simulink model "RoboticArmSimulation"  (R2025b)
settings: Solver=ode4  StartTime=0.0  StopTime=10  FixedStep=0.001  RelTol=1e-3
settings Model: Creator=james  LastModifiedBy=james

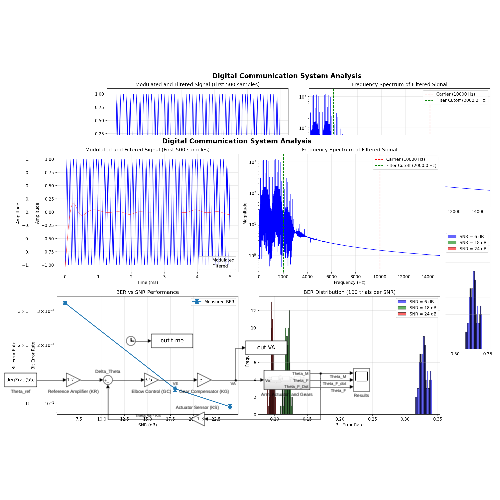
[thumbnail: Simulink's stored preview of the top-level diagram]
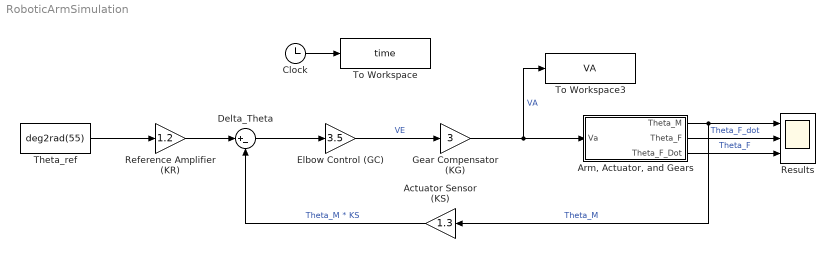
== system RoboticArmSimulation ==
  Actuator Sensor (KS) : Gain  Gain=1.3
  "Arm, Actuator, and Gears" : Subsystem
  Clock : Clock
  Delta_Theta : Sum  Inputs=|+-
  Elbow Control (GC) : Gain  Gain=3.5
  Gear Compensator (KG) : Gain  Gain=3
  Reference Amplifier (KR) : Gain  Gain=1.2
  Results : Scope  NumInputPorts=3
      settings: ActiveDisplayYMinimum=-2.9473768605800479  ActiveDisplayYMaximum=9.0057480309886788
  Theta_ref : Constant  Value=deg2rad(55)
  To Workspace : ToWorkspace  VariableName=time  SaveFormat=Timeseries  SampleTime=-1
  To Workspace3 : ToWorkspace  VariableName=VA  SaveFormat=Timeseries  SampleTime=-1
  wires:
  Theta_ref/1 -> Reference Amplifier (KR)/1
  Reference Amplifier (KR)/1 -> Delta_Theta/1
  Delta_Theta/1 -> Elbow Control (GC)/1
  Clock/1 -> To Workspace/1
  Elbow Control (GC)/1 -> Gear Compensator (KG)/1  "VE"
  Gear Compensator (KG)/1 -> To Workspace3/1, "Arm, Actuator, and Gears"/1(Va)  "VA"
  "Arm, Actuator, and Gears"/1(Theta_M) -> Actuator Sensor (KS)/1, Results/1  "Theta_M"
  "Arm, Actuator, and Gears"/2(Theta_F) -> Results/2  "Theta_F_dot"
  "Arm, Actuator, and Gears"/3(Theta_F_Dot) -> Results/3  "Theta_F"
  Actuator Sensor (KS)/1 -> Delta_Theta/2  "Theta_M * KS"

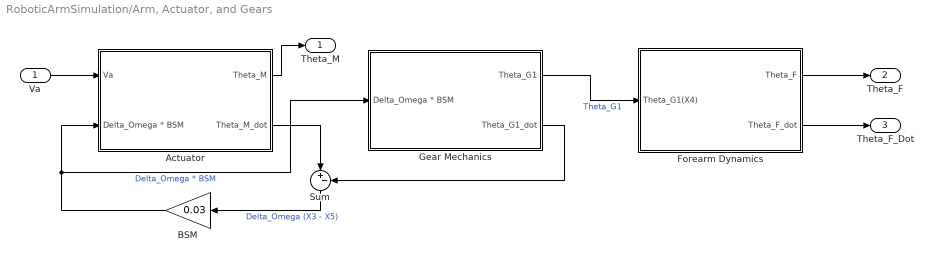
== system RoboticArmSimulation/Arm, Actuator, and Gears ==
  Va : Inport
  Actuator : Subsystem
  BSM : Gain  Gain=0.03
  Forearm Dynamics : Subsystem
  Gear Mechanics : Subsystem
  Sum : Sum  Inputs=|+-
  Theta_M : Outport
  Theta_F : Outport  Port=2
  Theta_F_Dot : Outport  Port=3
  wires:
  Va/1 -> Actuator/1(Va)
  Actuator/1(Theta_M) -> Theta_M/1
  Forearm Dynamics/1(Theta_F) -> Theta_F/1
  Forearm Dynamics/2(Theta_F_dot) -> Theta_F_Dot/1
  Gear Mechanics/1(Theta_G1) -> Forearm Dynamics/1(Theta_G1(X4))  "Theta_G1"
  Gear Mechanics/2(Theta_G1_dot) -> Sum/2
  Actuator/2(Theta_M_dot) -> Sum/1
  Sum/1 -> BSM/1  "Delta_Omega (X3 - X5)"
  BSM/1 -> Gear Mechanics/1(Delta_Omega * BSM), Actuator/2(Delta_Omega * BSM)  "Delta_Omega * BSM"

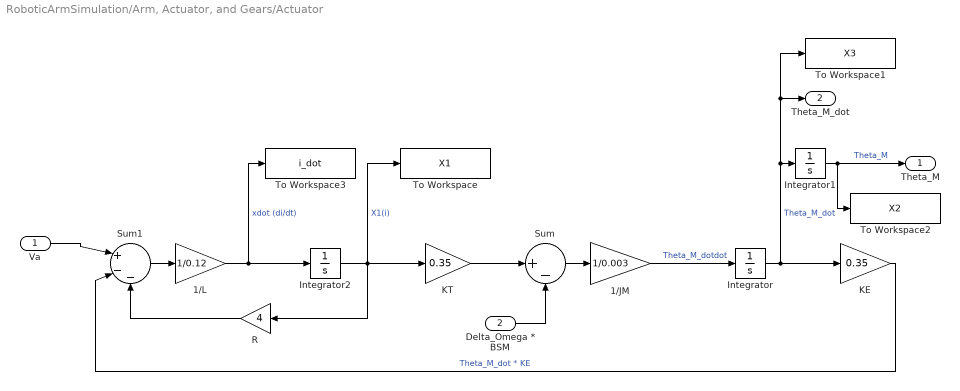
== system RoboticArmSimulation/Arm, Actuator, and Gears/Actuator ==
  Va : Inport
  Delta_Omega * BSM : Inport  Port=2
  1/JM : Gain  Gain=1/0.003
  1/L : Gain  Gain=1/0.12
  Integrator : Integrator
  Integrator1 : Integrator
  Integrator2 : Integrator
  KE : Gain  Gain=0.35
  KT : Gain  Gain=0.35
  R : Gain  Gain=4
  Sum : Sum  Inputs=|+-
  Sum1 : Sum  Inputs=|+--
  To Workspace : ToWorkspace  VariableName=X1  SaveFormat=Timeseries  SampleTime=-1
  To Workspace1 : ToWorkspace  VariableName=X3  SaveFormat=Timeseries  SampleTime=-1
  To Workspace2 : ToWorkspace  VariableName=X2  SaveFormat=Timeseries  SampleTime=-1
  To Workspace3 : ToWorkspace  VariableName=i_dot  SaveFormat=Timeseries  SampleTime=-1
  Theta_M : Outport
  Theta_M_dot : Outport  Port=2
  wires:
  Integrator2/1 -> To Workspace/1, KT/1, R/1  "X1(i)"
  KT/1 -> Sum/1
  Delta_Omega * BSM/1 -> Sum/2
  Sum/1 -> 1/JM/1
  1/JM/1 -> Integrator/1  "Theta_M_dotdot"
  Integrator/1 -> KE/1, To Workspace1/1, Theta_M_dot/1, Integrator1/1  "Theta_M_dot"
  KE/1 -> Sum1/2  "Theta_M_dot * KE"
  Integrator1/1 -> To Workspace2/1, Theta_M/1  "Theta_M"
  R/1 -> Sum1/3
  Va/1 -> Sum1/1
  Sum1/1 -> 1/L/1
  1/L/1 -> Integrator2/1, To Workspace3/1  "xdot (di/dt)"

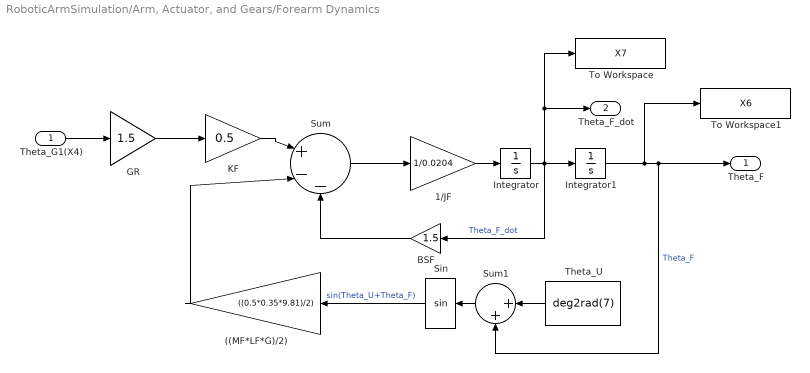
== system RoboticArmSimulation/Arm, Actuator, and Gears/Forearm Dynamics ==
  Theta_G1(X4) : Inport
  ((MF*LF*G)/2) : Gain  Gain=((0.5*0.35*9.81)/2)
  1/JF : Gain  Gain=1/0.0204
  BSF : Gain  Gain=1.5
  GR : Gain  Gain=1.5
  Integrator : Integrator
  Integrator1 : Integrator
  KF : Gain  Gain=0.5
  Sin : Trigonometry
  Sum : Sum  Inputs=|+--
  Sum1 : Sum  Inputs=|++
  Theta_U : Constant  Value=deg2rad(7)
  To Workspace : ToWorkspace  VariableName=X7  SaveFormat=Timeseries  SampleTime=-1
  To Workspace1 : ToWorkspace  VariableName=X6  SaveFormat=Timeseries  SampleTime=-1
  Theta_F : Outport
  Theta_F_dot : Outport  Port=2
  wires:
  Theta_G1(X4)/1 -> GR/1
  GR/1 -> KF/1
  KF/1 -> Sum/1
  Sum/1 -> 1/JF/1
  1/JF/1 -> Integrator/1
  Integrator/1 -> To Workspace/1, Theta_F_dot/1, Integrator1/1, BSF/1  "Theta_F_dot"
  Theta_U/1 -> Sum1/1
  Sin/1 -> ((MF*LF*G)/2)/1  "sin(Theta_U+Theta_F)"
  ((MF*LF*G)/2)/1 -> Sum/2
  Sum1/1 -> Sin/1
  Integrator1/1 -> Theta_F/1, Sum1/2, To Workspace1/1  "Theta_F"
  BSF/1 -> Sum/3

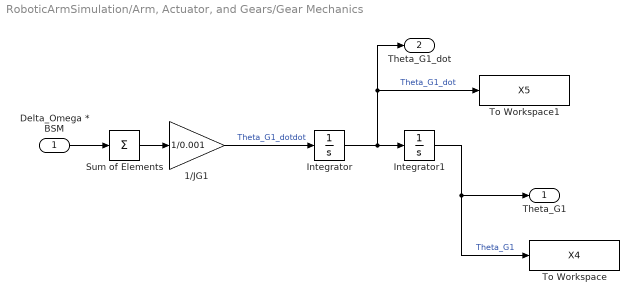
== system RoboticArmSimulation/Arm, Actuator, and Gears/Gear Mechanics ==
  Delta_Omega * BSM : Inport
  1/JG1 : Gain  Gain=1/0.001
  Integrator : Integrator
  Integrator1 : Integrator
  Sum of Elements : Sum  Inputs=+
  To Workspace : ToWorkspace  VariableName=X4  SaveFormat=Timeseries  SampleTime=-1
  To Workspace1 : ToWorkspace  VariableName=X5  SaveFormat=Timeseries  SampleTime=-1
  Theta_G1 : Outport
  Theta_G1_dot : Outport  Port=2
  wires:
  Delta_Omega * BSM/1 -> Sum of Elements/1
  1/JG1/1 -> Integrator/1  "Theta_G1_dotdot"
  Integrator/1 -> Integrator1/1, To Workspace1/1, Theta_G1_dot/1  "Theta_G1_dot"
  Integrator1/1 -> Theta_G1/1, To Workspace/1  "Theta_G1"
  Sum of Elements/1 -> 1/JG1/1
